simulink model "Fan"  (R2023a)
settings: Solver=VariableStepAuto  StartTime=0.0  StopTime=10.0  RelTol=1e-3  AbsTol=1e-3
model workspace (MAT data in the model file):
  Fan : object (value not decoded)
  Pipe : object (value not decoded)
libraries: fl_lib x10, nesl_utility x4, SimscapeFluids_lib x1
(part 3 of 3)

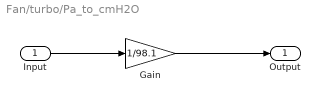
== system Fan/turbo/Pa_to_cmH2O ==
  Input : Inport
  Gain : Gain  Gain=1/98.1
  Output : Outport
  wires:
  Gain/1 -> Output/1
  Input/1 -> Gain/1

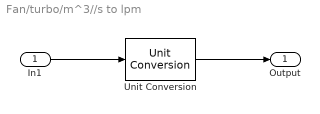
== system Fan/turbo/m^3//s to lpm  ==
  In1 : Inport  Unit=m^3/s
  Unit Conversion : UnitConversion
  Output : Outport  Unit=lpm
  wires:
  In1/1 -> Unit Conversion/1
  Unit Conversion/1 -> Output/1

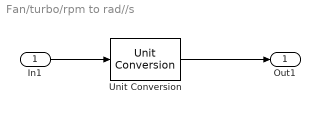
== system Fan/turbo/rpm to rad//s ==
  In1 : Inport  Unit=rpm
  Unit Conversion : UnitConversion
  Out1 : Outport  Unit=rad/s
  wires:
  In1/1 -> Unit Conversion/1
  Unit Conversion/1 -> Out1/1
